simulink model "synapse_spike_generator"  (R2020b)
settings: Solver=FixedStepDiscrete  StartTime=0.0  StopTime=stopTime  FixedStep=2.0833333333333333e-05  RelTol=1e-3
settings Model: Creator=Ross  LastModifiedBy=tyler
settings DataIOCC: SaveOutput=off  SaveTime=off  ReturnWorkspaceOutputs=off
settings OptimizationCC: BlockReduction=off  ConditionallyExecuteInputs=off  DefaultParameterBehavior=Inlined
settings DebuggingCC: ReadBeforeWriteMsg=DisableAll  WriteAfterWriteMsg=DisableAll  WriteAfterReadMsg=DisableAll  AlgebraicLoopMsg=error  MultiTaskDSMMsg=none  SingleTaskRateTransMsg=error  PregeneratedLibrarySubsystemCodeDiagnostic=none  ArithmeticOperatorsInVariantConditions=warning
settings HardwareCC: ProdBitPerPointer=32  ProdBitPerSizeT=32  ProdBitPerPtrDiffT=32  ProdLargestAtomicFloat=None  ProdIntDivRoundTo=Undefined  ProdEndianess=Unspecified  ProdWordSize=32  ProdHWDeviceType=ASIC/FPGA->ASIC/FPGA  TargetBitPerPointer=64  TargetBitPerSizeT=64  TargetBitPerPtrDiffT=64  TargetLongLongMode=on  TargetIntDivRoundTo=Zero  TargetEndianess=LittleEndian  TargetWordSize=64  TargetHWDeviceType=Custom Processor->MATLAB Host Computer  ProdEqTarget=off
settings ModelReferenceCC: UpdateModelReferenceTargets=IfOutOfDate  ModelReferenceNumInstancesAllowed=Single
settings SFSimCC: SFSimEcho=off  SimUseLocalCustomCode=off  CustomCodeUndefinedFunction=UseInterfaceOnly
settings RTWCC: RTWUseLocalCustomCode=off

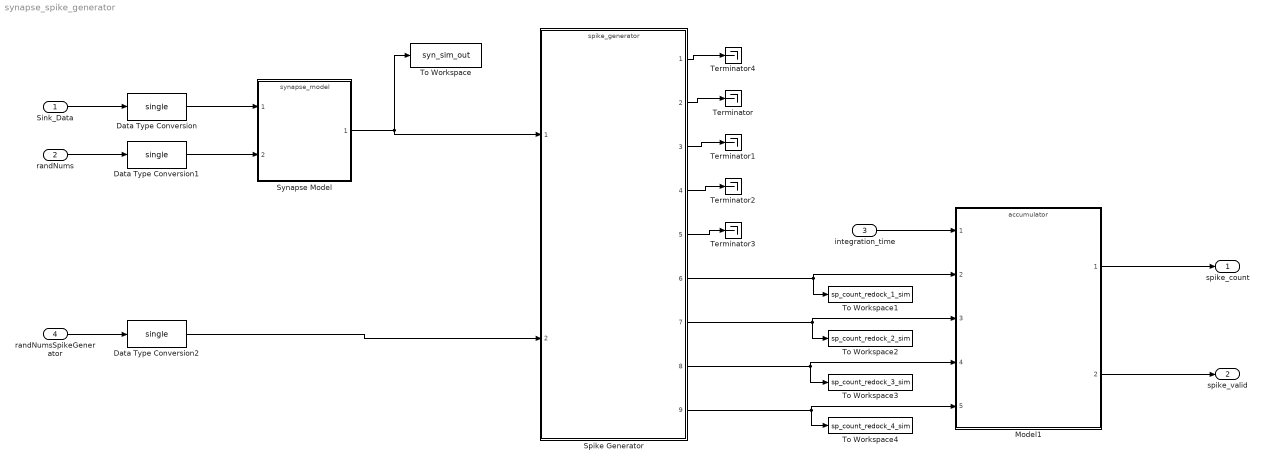
== system synapse_spike_generator ==
  Sink_Data : Inport  OutDataTypeStr=single  PortDimensions=1  SampleTime=[2.0833333333333333e-05,0]
  randNums : Inport  Port=2  OutDataTypeStr=single  PortDimensions=[1 1]  SampleTime=[2.0833333333333333e-05,0]
  integration_time : Inport  Port=3  OutDataTypeStr=uint32  PortDimensions=1  SampleTime=[2.0833333333333333e-05,0]
  randNumsSpikeGenerator : Inport  Port=4
  Data Type Conversion : DataTypeConversion  OutDataTypeStr=single
  Data Type Conversion1 : DataTypeConversion  OutDataTypeStr=single
  Data Type Conversion2 : DataTypeConversion  OutDataTypeStr=single
  Model1 : ModelReference  ModelNameDialog=accumulator  SimulationMode=Normal  ModelReferenceVersion=1.141
  Spike Generator : ModelReference  ModelNameDialog=spike_generator.slx  SimulationMode=Normal  ModelReferenceVersion=1.274
  Synapse Model : ModelReference  ModelNameDialog=synapse_model  SimulationMode=Normal  ModelReferenceVersion=1.138
  Terminator{,1..4} (5 alike) : Terminator
  To Workspace : ToWorkspace  VariableName=syn_sim_out  SampleTime=-1
  To Workspace1 : ToWorkspace  VariableName=sp_count_redock_1_sim  SampleTime=-1
  To Workspace2 : ToWorkspace  VariableName=sp_count_redock_2_sim  SampleTime=-1
  To Workspace3 : ToWorkspace  VariableName=sp_count_redock_3_sim  SampleTime=-1
  To Workspace4 : ToWorkspace  VariableName=sp_count_redock_4_sim  SampleTime=-1
  spike_count : Outport  OutDataTypeStr=fixdt(0,18,0)  PortDimensions=1  SampleTime=[2.0833333333333333e-05,0]
  spike_valid : Outport  Port=2  OutDataTypeStr=boolean  PortDimensions=1  SampleTime=[2.0833333333333333e-05,0]
  wires:
  Spike Generator/1 -> Terminator4/1
  Spike Generator/5 -> Terminator3/1
  Model1/1 -> spike_count/1
  Model1/2 -> spike_valid/1
  Spike Generator/2 -> Terminator/1
  Synapse Model/1 -> Spike Generator/1, To Workspace/1
  Sink_Data/1 -> Data Type Conversion/1
  Spike Generator/8 -> Model1/4, To Workspace3/1
  Spike Generator/9 -> Model1/5, To Workspace4/1
  Spike Generator/3 -> Terminator1/1
  Spike Generator/6 -> Model1/2, To Workspace1/1
  Data Type Conversion/1 -> Synapse Model/1
  Spike Generator/4 -> Terminator2/1
  integration_time/1 -> Model1/1
  Spike Generator/7 -> To Workspace2/1, Model1/3
  randNums/1 -> Data Type Conversion1/1
  Data Type Conversion1/1 -> Synapse Model/2
  randNumsSpikeGenerator/1 -> Data Type Conversion2/1
  Data Type Conversion2/1 -> Spike Generator/2
